simulink model "Practice6M"  (R2022a)
settings: Solver=ode113  StartTime=0.0  StopTime=10  MaxStep=1e-3  RelTol=1e-3
values from neighbouring files (symbols this model uses):
  A = [2,1;0,0]    [Practice6.m]
  B = [1;2]    [Practice6.m]
  C = [1,0]    [Practice6.m]
  K = double(Y)*P    [Practice6.m]
  L = P^(-1)*double(Y)    [Practice6.m]
settings Model: Creator=Administrator  LastModifiedBy=Administrator

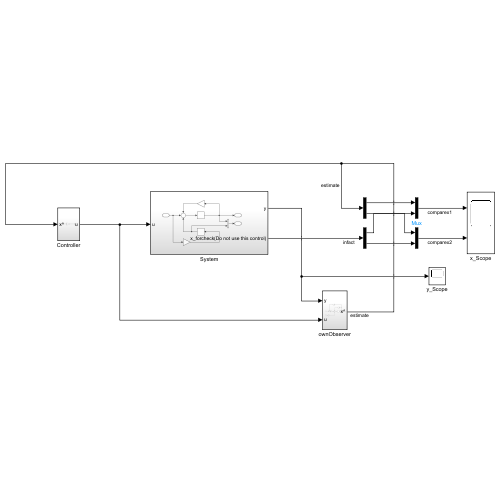
[thumbnail: Simulink's stored preview of the top-level diagram]
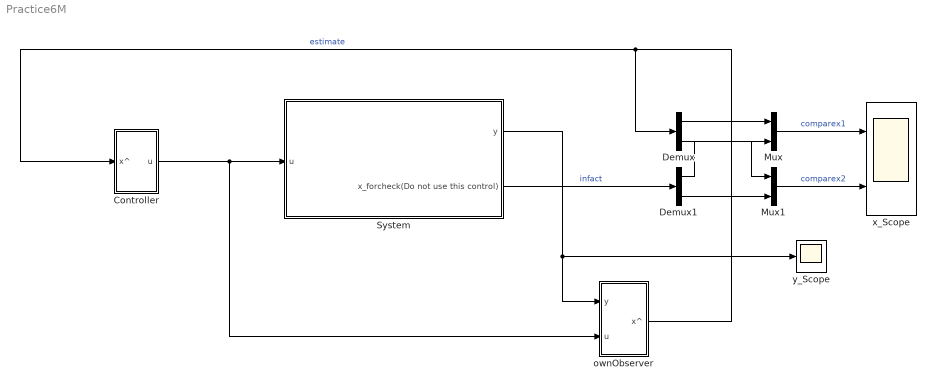
== system Practice6M ==
  Controller : Subsystem
  Demux : Demux  Outputs=2
  Demux1 : Demux  Outputs=2
  Mux : Mux  Inputs=2
  Mux1 : Mux  Inputs=2
  System : Subsystem
  ownObserver : Subsystem
  x_Scope : Scope  NumInputPorts=2
  y_Scope : Scope
  wires:
  Controller/1(u) -> ownObserver/2(u), System/1(u)
  System/1(y) -> y_Scope/1, ownObserver/1(y)
  ownObserver/1(x^) -> Demux/1, Controller/1(x^)  "estimate"
  System/2(x_forcheck(Do not use this control)) -> Demux1/1  "infact"
  Mux/1 -> x_Scope/1  "comparex1"
  Mux1/1 -> x_Scope/2  "comparex2"
  Demux1/2 -> Mux1/2
  Demux/2 -> Mux1/1
  Demux1/1 -> Mux/2
  Demux/1 -> Mux/1

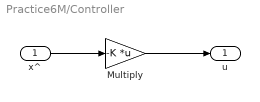
== system Practice6M/Controller ==
  x^ : Inport
  Multiply : Gain  Gain=-K  Multiplication=Matrix(K*u)
  u : Outport
  wires:
  Multiply/1 -> u/1
  x^/1 -> Multiply/1

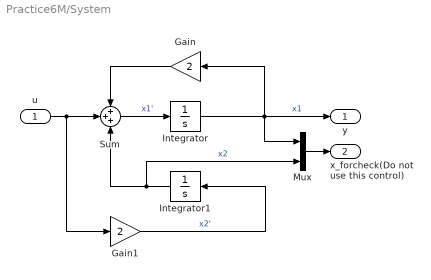
== system Practice6M/System ==
  u : Inport
  Gain : Gain  Gain=2
  Gain1 : Gain  Gain=2
  Integrator : Integrator  InitialCondition=3
  Integrator1 : Integrator  InitialCondition=5
  Mux : Mux  Inputs=2
  Sum : Sum  Inputs=+++
  y : Outport
  x_forcheck(Do not use this control) : Outport  Port=2
  wires:
  Integrator1/1 -> Mux/2, Sum/3  "x2"
  Gain/1 -> Sum/1
  Sum/1 -> Integrator/1  "x1'"
  Integrator/1 -> Mux/1, y/1, Gain/1  "x1"
  u/1 -> Gain1/1, Sum/2
  Gain1/1 -> Integrator1/1  "x2'"
  Mux/1 -> x_forcheck(Do not use this control)/1

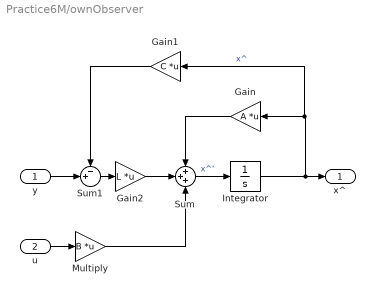
== system Practice6M/ownObserver ==
  y : Inport
  u : Inport  Port=2
  Gain : Gain  Gain=A  Multiplication=Matrix(K*u)
  Gain1 : Gain  Gain=C  Multiplication=Matrix(K*u)
  Gain2 : Gain  Gain=L  Multiplication=Matrix(K*u)
  Integrator : Integrator
  Multiply : Gain  Gain=B  Multiplication=Matrix(K*u)
  Sum : Sum  Inputs=+++
  Sum1 : Sum  Inputs=-+|
  x^ : Outport
  wires:
  Integrator/1 -> Gain1/1, Gain/1, x^/1  "x^"
  Sum/1 -> Integrator/1  "x^'"
  u/1 -> Multiply/1
  Multiply/1 -> Sum/3
  y/1 -> Sum1/2
  Gain/1 -> Sum/1
  Gain1/1 -> Sum1/1
  Sum1/1 -> Gain2/1
  Gain2/1 -> Sum/2
